simulink model "window_stateflow"  (R2025a)
settings: Solver=VariableStepAuto  StartTime=0.0  StopTime=10.0  RelTol=1e-3
settings Model: Creator=ISI  LastModifiedBy=ISI

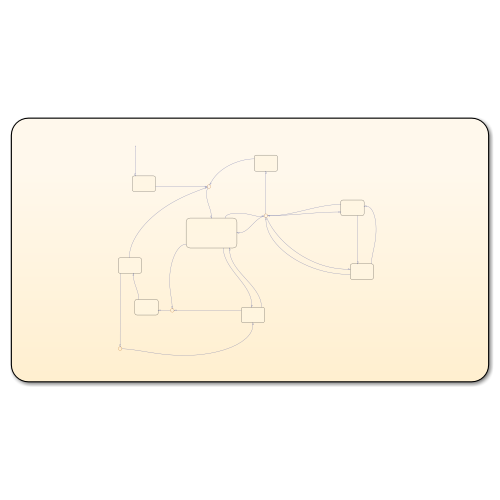
[thumbnail: Simulink's stored preview of the top-level diagram]
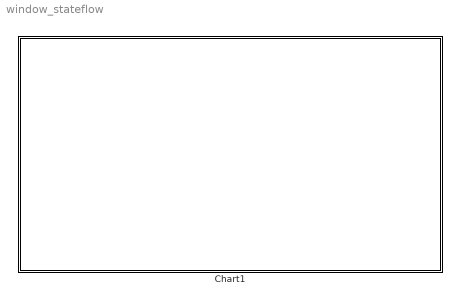
== system window_stateflow ==
  Chart1 : Stateflow chart  TreatAsAtomicUnit=on

== stateflow chart window_stateflow/Chart1 ==
  state Config
  state Init
  state Eph_Input
  state Standby
  state Waking_up
  state Manual
  state Sleep
  state Auto_Mode
  (default) -> Init : RESET
  Config -> (junction 160) : [end_submit]
  (junction 163) -> Config [order 2] : [begin_config]
  Init -> (junction 160) : [1]
  Waking_up -> (junction 160) [order 1] : [~auto_mode && data_loaded]
  (junction 160) -> Standby
  Eph_Input -> (junction 163) [order 1] : [end_eph_input]
  Manual -> Eph_Input [order 2] : [begin_eph_input]
  Standby -> (junction 163) [order 3]
  (junction 163) -> Eph_Input [order 3] : [begin_eph_input]
  Eph_Input -> Manual [order 2] : [begin_manual]
  (junction 163) -> Standby [order 1] : [1]
  (junction 163) -> Manual [order 4] : [begin_manual]
  Manual -> (junction 163) [order 1] : [end_manual]
  Standby -> (junction 164) [order 2]
  Standby -> Auto_Mode [order 1] : [toggle_auto_mode && ~auto_mode]
  Auto_Mode -> Standby [order 2] : [toggle_auto_mode && auto_mode]
  Waking_up -> Auto_Mode [order 2] : [auto_mode  && data_loaded]
  Sleep -> Waking_up : [wake_up]
  Auto_Mode -> (junction 164) [order 1]
  (junction 164) -> Sleep : [go_sleep]
  events: end_eph_input local FUNCTION_CALL_EVENT; begin_manual local FUNCTION_CALL_EVENT; begin_eph_input local FUNCTION_CALL_EVENT; begin_config local FUNCTION_CALL_EVENT; data_loaded local FUNCTION_CALL_EVENT; auto_mode local FUNCTION_CALL_EVENT; end_submit local FUNCTION_CALL_EVENT; end_manual local FUNCTION_CALL_EVENT; go_sleep local FUNCTION_CALL_EVENT; wake_up local FUNCTION_CALL_EVENT; toggle_auto_mode local FUNCTION_CALL_EVENT; RESET local FUNCTION_CALL_EVENT
